simulink model "chen_r2"  (Simulink 7.9)
settings: Solver=ode15s  StartTime=0.0  StopTime=60  FixedStep=0.001  RelTol=1e-3
values from neighbouring files (symbols this model uses):
  pc_p = Simulink.Parameter    [chen_init.m]
undefined symbols (not defined in the file or in its folder): pg
settings Model: Creator=toni  LastModifiedBy=toni  SimulationMode=rapid-accelerator  TunableVars=pc_p,pg_p  TunableVarsStorageClass=Auto,Auto  TunableVarsTypeQualifier=,
settings SFSimCC: SimParseCustomCode=off
settings GRTTargetCC: CombineOutputUpdateFcns=off  GRTInterface=on

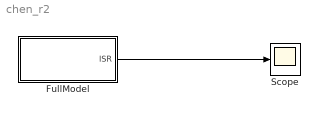
== system chen_r2 ==
  FullModel : Subsystem  mask{pc=<empty>}
      mask prompts: pc "Mask Parameter 1:"
      mask StyleString: popup(<empty>)
      mask TabNameString: Calcium
  Scope : Scope
      settings: YMin=0  YMax=225
  wires:
  FullModel/1(ISR) -> Scope/1

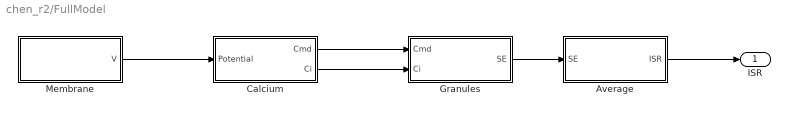
== system chen_r2/FullModel ==
  Average : Subsystem
  Calcium : Subsystem
  Granules : Subsystem
  Membrane : Subsystem
  ISR : Outport
  wires:
  Membrane/1(V) -> Calcium/1(Potential)
  Calcium/1(Cmd) -> Granules/1(Cmd)
  Calcium/2(Ci) -> Granules/2(Ci)
  Granules/1(SE) -> Average/1(SE)
  Average/1(ISR) -> ISR/1

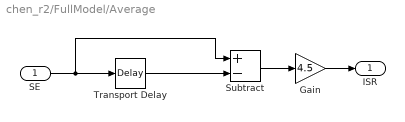
== system chen_r2/FullModel/Average ==
  SE : Inport
  Gain : Gain  Gain=4.5
  Subtract : Sum  Inputs=+-
  Transport Delay : TransportDelay  DelayTime=2
  ISR : Outport
  wires:
  SE/1 -> Transport Delay/1, Subtract/1
  Transport Delay/1 -> Subtract/2
  Subtract/1 -> Gain/1
  Gain/1 -> ISR/1

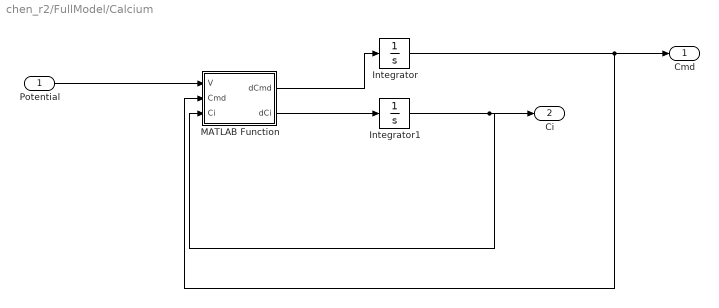
== system chen_r2/FullModel/Calcium ==
  Potential : Inport
  Integrator : Integrator  InitialCondition=pc_p.Cmd0
  Integrator1 : Integrator  InitialCondition=pc_p.Ci0
  MATLAB Function : MATLAB Function  TreatAsAtomicUnit=on
  Cmd : Outport
  Ci : Outport  Port=2
  wires:
  Integrator/1 -> MATLAB Function/2(Cmd), Cmd/1
  Integrator1/1 -> MATLAB Function/3(Ci), Ci/1
  MATLAB Function/2(dCi) -> Integrator1/1
  MATLAB Function/1(dCmd) -> Integrator/1
  Potential/1 -> MATLAB Function/1(V)

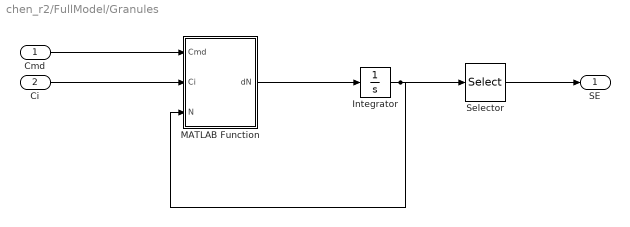
== system chen_r2/FullModel/Granules ==
  Cmd : Inport
  Ci : Inport  Port=2
  Integrator : Integrator  InitialCondition=pg.N_0
  MATLAB Function : MATLAB Function  TreatAsAtomicUnit=on
  Selector : Selector  InputPortWidth=9  IndexOptions=Index vector (dialog)  Indices=9  OutputSizes=1
  SE : Outport
  wires:
  MATLAB Function/1(dN) -> Integrator/1
  Integrator/1 -> MATLAB Function/3(N), Selector/1
  Ci/1 -> MATLAB Function/2(Ci)
  Cmd/1 -> MATLAB Function/1(Cmd)
  Selector/1 -> SE/1

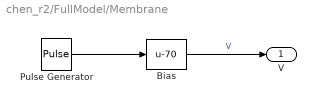
== system chen_r2/FullModel/Membrane ==
  Bias : Bias  Bias=-70
  Pulse Generator : DiscretePulseGenerator  PulseType=Time based  Amplitude=50  Period=12  PulseWidth=50
  V : Outport
  wires:
  Pulse Generator/1 -> Bias/1
  Bias/1 -> V/1  "V"

== matlab function FullModel/Granules/MATLAB Function ==
  data: Cmd input double; dN output double; Ci input double; N input double; pg_p parameter double
function dN = fcn(Cmd,Ci,N,pg_p)
%#codegen

% N is the granule populations.
%  N(1) .. N(6) are N1..N6, NF, NR, SE

    dN=zeros(9,1);

    r2 = pg_p.r20*Ci/(Ci + pg_p.Kp2);
    r3 = pg_p.GlucFact*pg_p.r30*Ci/(Ci + pg_p.Kp);

        % shortcuts
    N1=N(1); N2=N(2); N3=N(3); N4=N(4); N5=N(5); N6=N(6); 
    NF=N(7); NR=N(8); 
    
        %shortcuts
    k1=pg_p.k1;
    km1=pg_p.km1;
    r1=pg_p.r1;
    rm1=pg_p.rm1;
    rm2=pg_p.rm2;
    rm3=pg_p.rm3; 
    u1=pg_p.u1; 
    u2=pg_p.u2; 
    u3=pg_p.u3;

    
    dN(1) = pg_p.ts*(-(3*k1*Cmd + rm1)*N1 + km1*N2 + r1*N5);		% Primed
    dN(2) = pg_p.ts*(3*k1*Cmd*N1 -(2*k1*Cmd + km1)*N2 + 2*km1*N3); 	% Bound
    dN(3) = pg_p.ts*(2*k1*Cmd*N2 -(2*km1 + k1*Cmd)*N3 + 3*km1*N4); 	% Triggered
    dN(4) = pg_p.ts*(k1*Cmd*N3 - (3*km1 + u1)*N4); 	   		% Fused
    dN(5) = pg_p.ts*(rm1*N1 - (r1 + rm2)*N5 + r2*N6); 		% Primed
    dN(6) = pg_p.ts*(r3 + rm2*N5 - (rm3 + r2)*N6); 			% Docked
    dN(7) = pg_p.ts*(u1*N4 - u2*NF);      				% Fused
    dN(8) = pg_p.ts*(u2*NF - u3*NR); 				% Releasing
    dN(9) = pg_p.ts*(u3*NR); 					% Secretion



end

== matlab function FullModel/Calcium/MATLAB Function ==
  data: V input double; Cmd input double; Ci input double; dCmd output double; pc_p parameter double; dCi output double
function [dCmd, dCi] = fcn(V, Cmd, Ci, pc_p)
%#codegen

    Jserca = pc_p.Jsercamax*Ci^2/(pc_p.Kserca^2 + Ci^2);
    Jpmca  = pc_p.Jpmcamax*Ci/(pc_p.Kpmca + Ci);
    Jncx   = pc_p.Jncx0*(Ci - 0.25);
    L = Jserca + Jpmca + Jncx + pc_p.Jleak;

    
    IL = pc_p.gL*minf(V,pc_p.Vm,pc_p.sm)*(V-pc_p.Vca);
    IR = 0.25*IL;

    JL = pc_p.alpha*IL/pc_p.vmd;
    JR = pc_p.alpha*IR/pc_p.vcell;

    dCmd = pc_p.ts*(-pc_p.fmd*JL - pc_p.fmd*pc_p.B*(Cmd - Ci));
    dCi =  pc_p.ts*(-pc_p.fi*JR  + pc_p.fv*pc_p.fi*pc_p.B*(Cmd - Ci) - pc_p.fi*L);

end      
    
function out=minf(V,Vm,sm)
%#codegen
    out=    1/(1 + exp((Vm-V)/sm));
end
